simulink model "mi_simuladorControlCuatrirrotor"  (Simulink 8.0)
settings: Solver=ode45  StartTime=0.0  StopTime=720  FixedStep=0.06  MaxStep=0.06  RelTol=1e-3
values from neighbouring files (symbols this model uses):
  radio = 0.1    [simulaControl.m]
  ruta = [0,0;ruta]    [pintascdata.m]    (also in pintascdata_tb2.m; simulaControl.m = [12 12;12 12])
undefined symbols (not defined in the file or in its folder): DiscIntNeverNeededParam, Ts
libraries: simulink x7, slident x2
settings Model: Creator=xblasco  LastModifiedBy=Elisa
settings DataIOCC: SignalLoggingSaveFormat=ModelDataLogs
settings DebuggingCC: FcnCallInpInsideContextMsg=UseLocalSettings  StrictBusMsg=Warning
settings GRTTargetCC: CombineOutputUpdateFcns=off  GRTInterface=on

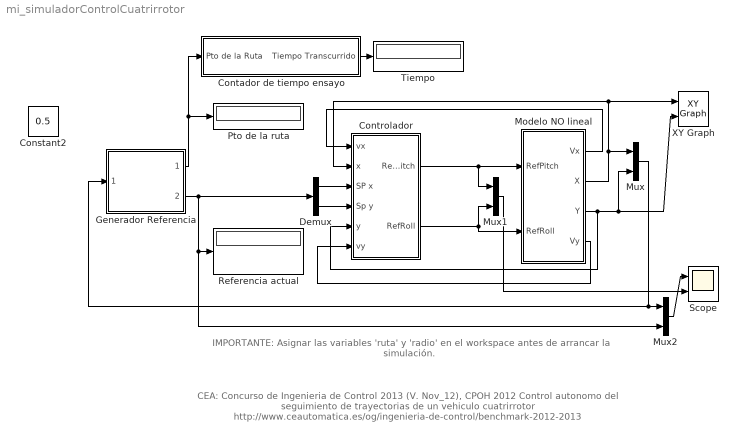
== system mi_simuladorControlCuatrirrotor ==
  note: IMPORTANTE:
      | Asignar las variables 'ruta' y 'radio' en el workspace antes de arrancar la simulación.
  note: CEA: Concurso de Ingenieria de Control 2013 (V. Nov_12), CPOH 2012
      | Control autonomo del seguimiento de trayectorias de un vehiculo cuatrirrotor
      | http://www.ceautomatica.es/og/ingenieria-de-control/benchmark-2012-2013
  " Modelo NO lineal" : Subsystem
  Contador de tiempo ensayo : Subsystem
  Controlador : Subsystem
  Demux : Demux  Outputs=2
  Generador Referencia : Subsystem
  Mux : Mux  Inputs=2
  Mux1 : Mux  Inputs=2
  Mux2 : Mux  Inputs=2
  Pto de la ruta : Display
  Referencia actual : Display
  Scope : Scope  NumInputPorts=2
      settings: YMin=-5~-1  YMax=15~1  SaveName=scdata  SampleInput=on  SampleTime=0.06
  Tiempo : Display
  XY Graph : simulink/Sinks/XY Graph  xmin=-10  xmax=15  ymin=-6  ymax=6  st=-1
  Constant2 : Constant  IOType=siggen  Value=0.5
  wires:
  Generador Referencia/2(Siguiente pos) -> Mux2/2, Referencia actual/1, Demux/1
  Generador Referencia/1(Pto de la ruta) -> Pto de la ruta/1, Contador de tiempo ensayo/1(Pto de la Ruta)
  Mux/1 -> Generador Referencia/1(Posicion  actual), Mux2/1
  Controlador/2(RefRoll) -> " Modelo NO lineal"/2(RefRoll), Mux1/2
  Controlador/1(RefPitch) -> " Modelo NO lineal"/1(RefPitch), Mux1/1
  " Modelo NO lineal"/2(X) -> Mux/1, XY Graph/1, Controlador/2(x)
  Mux1/1 -> Scope/2
  " Modelo NO lineal"/1(Vx) -> Controlador/1(vx)
  Mux2/1 -> Scope/1
  Demux/1 -> Controlador/3(SP x)
  Demux/2 -> Controlador/4(Sp y)
  Contador de tiempo ensayo/1(Tiempo Transcurrido) -> Tiempo/1
  " Modelo NO lineal"/3(Y) -> Mux/2, XY Graph/2, Controlador/5(y)
  " Modelo NO lineal"/4(Vy) -> Controlador/6(vy)

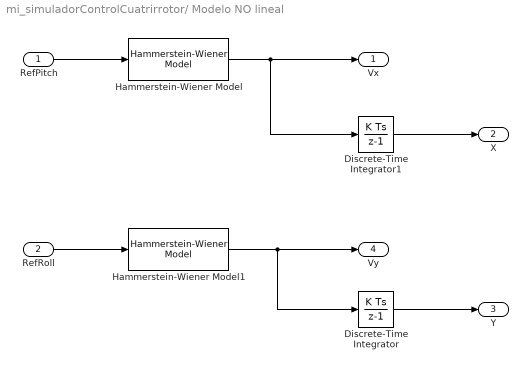
== system mi_simuladorControlCuatrirrotor/ Modelo NO lineal ==
  RefPitch : Inport  PortDimensions=1  SampleTime=0.06
  RefRoll : Inport  Port=2  PortDimensions=1  SampleTime=0.06
  Discrete-Time Integrator : DiscreteIntegrator  SampleTime=Ts  ICPrevOutput=DiscIntNeverNeededParam  ICPrevScaledInput=DiscIntNeverNeededParam
  Discrete-Time Integrator1 : DiscreteIntegrator  SampleTime=Ts  ICPrevOutput=DiscIntNeverNeededParam  ICPrevScaledInput=DiscIntNeverNeededParam
  Hammerstein-Wiener Model : slident/Hammerstein-Wiener Model  sys=vx123_nlhw122bis  IC=Zero  X0i=0
  Hammerstein-Wiener Model1 : slident/Hammerstein-Wiener Model  sys=vy123_nlhw111  IC=Zero  X0i=0
  Vx : Outport
  X : Outport  Port=2
  Y : Outport  Port=3
  Vy : Outport  Port=4
  wires:
  Hammerstein-Wiener Model1/1 -> Discrete-Time Integrator/1, Vy/1
  Hammerstein-Wiener Model/1 -> Discrete-Time Integrator1/1, Vx/1
  RefRoll/1 -> Hammerstein-Wiener Model1/1
  RefPitch/1 -> Hammerstein-Wiener Model/1
  Discrete-Time Integrator/1 -> Y/1
  Discrete-Time Integrator1/1 -> X/1

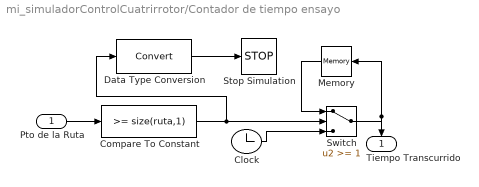
== system mi_simuladorControlCuatrirrotor/Contador de tiempo ensayo ==
  Pto de la Ruta : Inport
  Clock : Clock
  Compare To Constant : simulink/Logic and Bit Operations/Compare To Constant  relop=>=  const=size(ruta,1)  OutDataTypeStr=uint8
  Data Type Conversion : DataTypeConversion
  Memory : Memory
  Stop Simulation : Stop
  Switch : Switch  Threshold=1
  Tiempo Transcurrido : Outport
  wires:
  Clock/1 -> Switch/3
  Compare To Constant/1 -> Switch/2, Data Type Conversion/1
  Switch/1 -> Memory/1, Tiempo Transcurrido/1
  Memory/1 -> Switch/1
  Data Type Conversion/1 -> Stop Simulation/1
  Pto de la Ruta/1 -> Compare To Constant/1

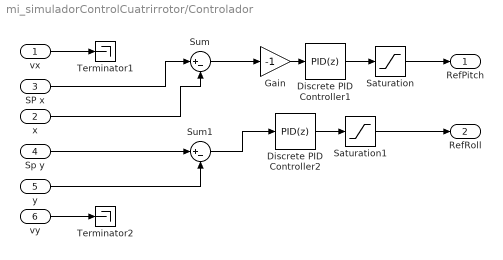
== system mi_simuladorControlCuatrirrotor/Controlador ==
  vx : Inport
  x : Inport  Port=2
  SP x : Inport  Port=3
  Sp y : Inport  Port=4
  y : Inport  Port=5
  vy : Inport  Port=6
  Discrete PID Controller1 : simulink/Continuous/PID Controller  Controller=PID  TimeDomain=Discrete-time  SampleTime=Ts  IntegratorMethod=Forward Euler  FilterMethod=Forward Euler  Form=Parallel  P=0.7  I=0  D=0.5  N=15  InitialConditionSource=internal  InitialConditionForIntegrator=0  InitialConditionForFilter=0  ExternalReset=none  LimitOutput=off  UpperSaturationLimit=inf  LowerSaturationLimit=-inf  LinearizeAsGain=off  AntiWindupMode=none  Kb=1  TrackingMode=off  Kt=1  PParamMin=[]  PParamMax=[]  IParamMin=[]  IParamMax=[]  DParamMin=[]  DParamMax=[]  NParamMin=[]  NParamMax=[]  KbParamMin=[]  KbParamMax=[]  KtParamMin=[]  KtParamMax=[]  POutMin=[]  POutMax=[]  IOutMin=[]  IOutMax=[]  DOutMin=[]  DOutMax=[]  NOutMin=[]  NOutMax=[]  KbOutMin=[]  KbOutMax=[]  KtOutMin=[]  KtOutMax=[]  IntegratorOutMin=[]  IntegratorOutMax=[]  FilterOutMin=[]  FilterOutMax=[]  SumOutMin=[]  SumOutMax=[]  SumI1OutMin=[]  SumI1OutMax=[]  SumI2OutMin=[]  SumI2OutMax=[]  SumI3OutMin=[]  SumI3OutMax=[]  SumDOutMin=[]  SumDOutMax=[]  SaturationOutMin=[]  SaturationOutMax=[]  IntegratorContinuousStateAttributes=''  IntegratorStateMustResolveToSignalObject=off  IntegratorRTWStateStorageClass=Auto  FilterContinuousStateAttributes=''  FilterStateMustResolveToSignalObject=off  FilterRTWStateStorageClass=Auto
  Discrete PID Controller2 : simulink/Continuous/PID Controller  Controller=PID  TimeDomain=Discrete-time  SampleTime=Ts  IntegratorMethod=Forward Euler  FilterMethod=Forward Euler  Form=Parallel  P=1.6  I=0  D=0.7  N=8  InitialConditionSource=internal  InitialConditionForIntegrator=0  InitialConditionForFilter=0  ExternalReset=none  LimitOutput=off  UpperSaturationLimit=inf  LowerSaturationLimit=-inf  LinearizeAsGain=off  AntiWindupMode=none  Kb=1  TrackingMode=off  Kt=1  PParamMin=[]  PParamMax=[]  IParamMin=[]  IParamMax=[]  DParamMin=[]  DParamMax=[]  NParamMin=[]  NParamMax=[]  KbParamMin=[]  KbParamMax=[]  KtParamMin=[]  KtParamMax=[]  POutMin=[]  POutMax=[]  IOutMin=[]  IOutMax=[]  DOutMin=[]  DOutMax=[]  NOutMin=[]  NOutMax=[]  KbOutMin=[]  KbOutMax=[]  KtOutMin=[]  KtOutMax=[]  IntegratorOutMin=[]  IntegratorOutMax=[]  FilterOutMin=[]  FilterOutMax=[]  SumOutMin=[]  SumOutMax=[]  SumI1OutMin=[]  SumI1OutMax=[]  SumI2OutMin=[]  SumI2OutMax=[]  SumI3OutMin=[]  SumI3OutMax=[]  SumDOutMin=[]  SumDOutMax=[]  SaturationOutMin=[]  SaturationOutMax=[]  IntegratorContinuousStateAttributes=''  IntegratorStateMustResolveToSignalObject=off  IntegratorRTWStateStorageClass=Auto  FilterContinuousStateAttributes=''  FilterStateMustResolveToSignalObject=off  FilterRTWStateStorageClass=Auto
  Gain : Gain  Gain=-1  SampleTime=Ts
  Saturation : Saturate  UpperLimit=0.3  LowerLimit=-0.3  SampleTime=Ts
  Saturation1 : Saturate  UpperLimit=1  LowerLimit=-1  SampleTime=Ts
  Sum : Sum  Inputs=|+-
  Sum1 : Sum  Inputs=|+-
  Terminator1 : Terminator
  Terminator2 : Terminator
  RefPitch : Outport
  RefRoll : Outport  Port=2
  wires:
  Sum1/1 -> Discrete PID Controller2/1
  Saturation/1 -> RefPitch/1
  x/1 -> Sum/2
  SP x/1 -> Sum/1
  vx/1 -> Terminator1/1
  vy/1 -> Terminator2/1
  y/1 -> Sum1/2
  Sp y/1 -> Sum1/1
  Sum/1 -> Gain/1
  Gain/1 -> Discrete PID Controller1/1
  Discrete PID Controller1/1 -> Saturation/1
  Discrete PID Controller2/1 -> Saturation1/1
  Saturation1/1 -> RefRoll/1

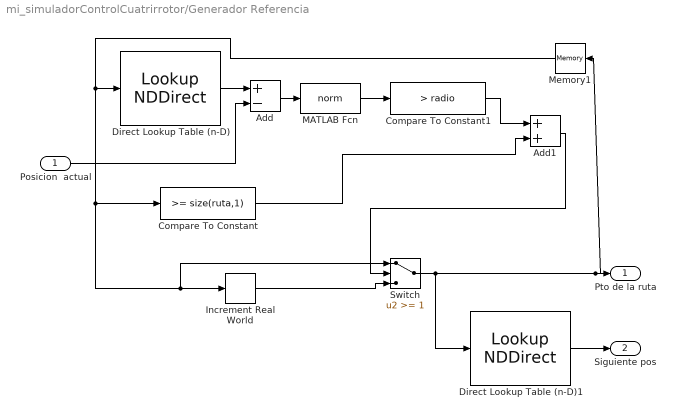
== system mi_simuladorControlCuatrirrotor/Generador Referencia ==
  Posicion  actual : Inport
  Add : Sum  Inputs=+-
  Add1 : Sum
  Compare To Constant : simulink/Logic and Bit Operations/Compare To Constant  relop=>=  const=size(ruta,1)  OutDataTypeStr=uint8
  Compare To Constant1 : simulink/Logic and Bit Operations/Compare To Constant  relop=>  const=radio  OutDataTypeStr=uint8
  Direct Lookup Table (n-D) : LookupNDDirect  InputsSelectThisObjectFromTable=Column  Table=ruta'
  Direct Lookup Table (n-D)1 : LookupNDDirect  InputsSelectThisObjectFromTable=Column  Table=ruta'
  Increment Real World : simulink/Additional Math & Discrete/Additional Math: Increment - Decrement/Increment Real World
  MATLAB Fcn : MATLABFcn  MATLABFcn=norm  Output1D=off
  Memory1 : Memory
  Switch : Switch  Threshold=1
  Pto de la ruta : Outport
  Siguiente pos : Outport  Port=2
  wires:
  Direct Lookup Table (n-D)/1 -> Add/1
  Add/1 -> MATLAB Fcn/1
  Increment Real World/1 -> Switch/3
  Switch/1 -> Direct Lookup Table (n-D)1/1, Pto de la ruta/1, Memory1/1
  Posicion  actual/1 -> Add/2
  Direct Lookup Table (n-D)1/1 -> Siguiente pos/1
  MATLAB Fcn/1 -> Compare To Constant1/1
  Compare To Constant1/1 -> Add1/1
  Compare To Constant/1 -> Add1/2
  Add1/1 -> Switch/2
  Memory1/1 -> Direct Lookup Table (n-D)/1, Switch/1, Increment Real World/1, Compare To Constant/1
